simulink model "w3p2"  (R2020b)
settings: Solver=VariableStepAuto  StartTime=0.0  StopTime=10.0  RelTol=1e-3
undefined symbols (not defined in the file): DiscIntNeverNeededParam
libraries: simulink x1
settings Model: Creator=WELCOME  LastModifiedBy=WELCOME

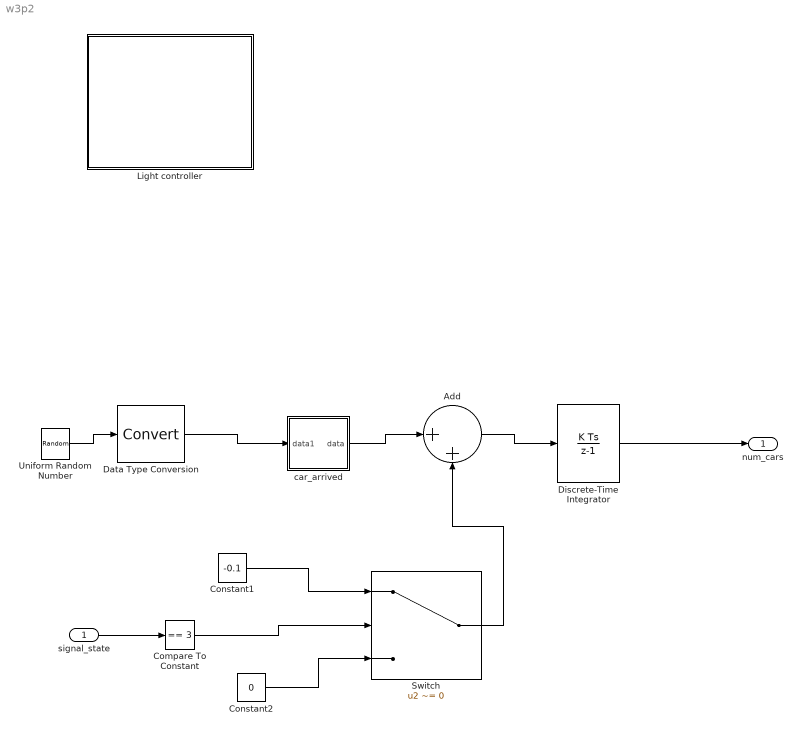
== system w3p2 ==
  signal_state : Inport
  Add : Sum  Inputs=|++
  Compare To Constant : simulink/Logic and Bit Operations/Compare To Constant  relop===  const=3  OutDataTypeStr=boolean  ZeroCross=off
  Constant1 : Constant  Value=-0.1
  Constant2 : Constant  Value=0
  Data Type Conversion : DataTypeConversion
  Discrete-Time Integrator : DiscreteIntegrator  SampleTime=-1  LimitOutput=on  LowerSaturationLimit=0  ICPrevOutput=DiscIntNeverNeededParam  ICPrevScaledInput=DiscIntNeverNeededParam
  Light controller : Stateflow chart  TreatAsAtomicUnit=on
  Switch : Switch  Criteria=u2 ~= 0
  Uniform Random Number : UniformRandomNumber  Minimum=0  Maximum=100  Seed=177836  SampleTime=0
  car_arrived : Stateflow chart  TreatAsAtomicUnit=on
  num_cars : Outport  VectorParamsAs1DForOutWhenUnconnected=off
  wires:
  Add/1 -> Discrete-Time Integrator/1
  Discrete-Time Integrator/1 -> num_cars/1
  car_arrived/1(data) -> Add/1
  Data Type Conversion/1 -> car_arrived/1(data1)
  Uniform Random Number/1 -> Data Type Conversion/1
  Constant1/1 -> Switch/1
  Compare To Constant/1 -> Switch/2
  Constant2/1 -> Switch/3
  signal_state/1 -> Compare To Constant/1
  Switch/1 -> Add/2

== stateflow chart w3p2/car_arrived ==
  (default) -> (junction 2) : {out = in > 98;}
  data: data output; data1 input

== stateflow chart w3p2/Light controller ==
  state Stop
    y1=RED;
    y2=GREEN;
  state StopForTraffic
    y1=RED;
    y2=GREEN;
  state StoptoGo
    y1=RED;
    y2=YELLOW;
  state GoToStop
    y1=YELLOW;
    y2=RED;
  state Go
    y1=GREEN;
    y2=RED;
  (default) -> Stop
  Stop -> StopForTraffic : after(20,tick)
  StopForTraffic -> StoptoGo : [sens]
  GoToStop -> Stop : after(3,tick)
  StoptoGo -> Go : after(3,tick)
  Go -> GoToStop : after(10,tick)
